simulink model "mypid"  (R2016a)
settings: Solver=VariableStepAuto  StartTime=0.0  StopTime=10.0  RelTol=1e-3
settings Model: SnapshotBufferSize=1  Creator=Shinelon  LastModifiedBy=Shinelon

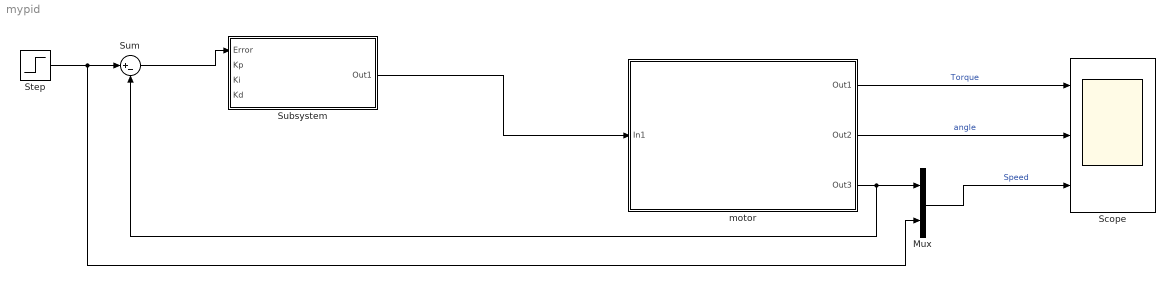
== system mypid ==
  Mux : Mux  Inputs=2
  Scope : Scope  NumInputPorts=3
  Step : Step  Time=5  After=100  SampleTime=0
  Subsystem : Subsystem
  Sum : Sum  Inputs=|+-
  "motor " : Subsystem  mask(DC motor subsystem){R=2, L=0.5, Km=0.1, Kf=0.2, Kemf=0.1, J=0.02}
      mask prompts: R "Resistor"; L "Inductor"; Km "Torque Constant"; Kf "Viscous Friction Constant"; Kemf "Back EMF Votage Constant"; J "Inertial Load"
      mask help:
      | This is a DC motor subsystem
      | Input : Control Signal
      | Output : Motor Rate
      mask init:
      | R=2;
      | L=0.5;
      | Km=0.1;
      | Kemf=0.1;
      | Kf=0.2;
      | J=0.02;
      mask Display:
      | color('red');port_label('input',1,'Control Signal');
      | color('red');port_label('output',1,'Torque');
      | color('red');port_label('output',2,'Angle');
      | color('red');port_label('output',3,'Speed');
      | image(imread('E:\simulink model\DC motor model\timg.jpg'))
  wires:
  Mux/1 -> Scope/3  "Speed"
  "motor "/1(Out1) -> Scope/1  "Torque"
  "motor "/2(Out2) -> Scope/2  "angle"
  "motor "/3(Out3) -> Sum/2, Mux/1
  Step/1 -> Mux/2, Sum/1
  Sum/1 -> Subsystem/1("Error ")
  Subsystem/1(Out1) -> "motor "/1(In1)

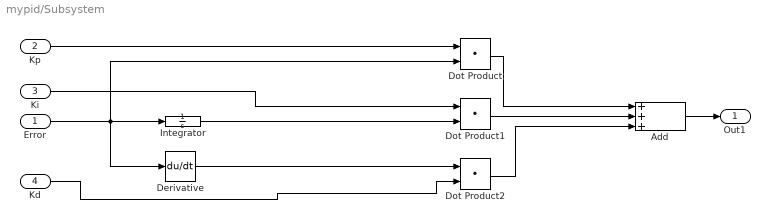
== system mypid/Subsystem ==
  "Error " : Inport
  "Kp " : Inport  Port=2
  "Ki " : Inport  Port=3
  Kd : Inport  Port=4
  Add : Sum  Inputs=+++
  Derivative : Derivative
  Dot Product : DotProduct  InputSameDT=on  OutDataTypeStr=Inherit: Inherit via internal rule
  Dot Product1 : DotProduct  InputSameDT=on  OutDataTypeStr=Inherit: Inherit via internal rule
  Dot Product2 : DotProduct  InputSameDT=on  OutDataTypeStr=Inherit: Inherit via internal rule
  Integrator : Integrator
  Out1 : Outport
  wires:
  Integrator/1 -> Dot Product1/2
  Dot Product2/1 -> Add/3
  "Error "/1 -> Dot Product/2, Integrator/1, Derivative/1
  Derivative/1 -> Dot Product2/1
  Dot Product/1 -> Add/1
  "Ki "/1 -> Dot Product1/1
  Add/1 -> Out1/1
  Kd/1 -> Dot Product2/2
  Dot Product1/1 -> Add/2
  "Kp "/1 -> Dot Product/1

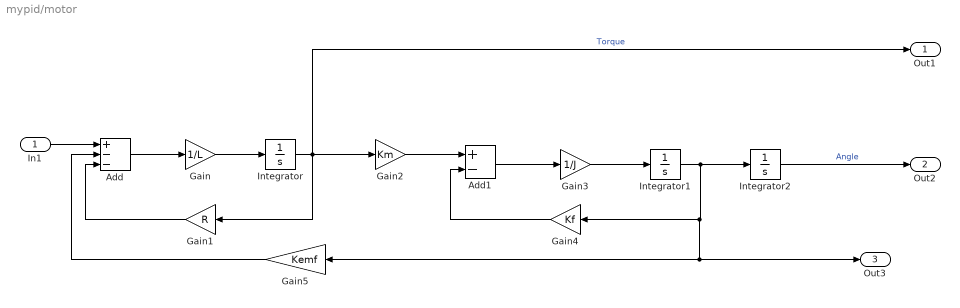
== system mypid/motor  ==
  In1 : Inport
  Add : Sum  Inputs=+--
  Add1 : Sum  Inputs=+-
  Gain : Gain  Gain=1/L
  Gain1 : Gain  Gain=R
  Gain2 : Gain  Gain=Km
  Gain3 : Gain  Gain=1/J
  Gain4 : Gain  Gain=Kf
  Gain5 : Gain  Gain=Kemf
  Integrator : Integrator
  Integrator1 : Integrator
  Integrator2 : Integrator
  Out1 : Outport
  Out2 : Outport  Port=2
  Out3 : Outport  Port=3
  wires:
  Gain5/1 -> Add/2
  Integrator/1 -> Out1/1, Gain2/1, Gain1/1  "Torque"
  Integrator2/1 -> Out2/1  "Angle"
  Add/1 -> Gain/1
  Gain/1 -> Integrator/1
  Gain1/1 -> Add/3
  Gain2/1 -> Add1/1
  Add1/1 -> Gain3/1
  Gain3/1 -> Integrator1/1
  Integrator1/1 -> Integrator2/1, Out3/1, Gain5/1, Gain4/1
  Gain4/1 -> Add1/2
  In1/1 -> Add/1
